simulink model "Symmetry"  (Simulink 8.3)
settings: Solver=ode23t  StartTime=0.0  StopTime=tfin  RelTol=1e-4
values from neighbouring files (symbols this model uses):
  Butterworth_filter_order = 8    [Sketch_controller_model_ini.m]    (also in Symmetry_ini.m; Symmetry_ini_COPY.m)
  C_Network = [0, 0, 0]    [Symmetry_ini.m]    (also in Symmetry_ini_COPY.m)
  Capacitive_Load_R_RC = [25,    50,   35;                                10e-3, 5e-3, 7e-3]    [Symmetry_ini.m]    (also in Symmetry_ini_COPY.m = [60e-3,  120e-3,  80e-3;                                1e-3)
  Capacitive_Load_R_Switching_Sequence = Capacitive_Load_R_Switching_Sequence_'    [Symmetry_ini.m]    (also in Symmetry_ini_COPY.m = ones(3,tfin/Capacitive_Load_R_Switching_Speed(1))')
  Capacitive_Load_R_Switching_Speed = [0.02,0.02,0.02]    [Symmetry_ini.m]    (also in Symmetry_ini_COPY.m = [0.01,0.01,0.01])
  Capacitive_Load_S_RC = [25,    50,   35;                                10e-3, 5e-3, 7e-3]    [Symmetry_ini.m]    (also in Symmetry_ini_COPY.m = [60e-3,  120e-3,  80e-3;                                1e-3)
  Capacitive_Load_S_Switching_Sequence = Capacitive_Load_S_Switching_Sequence_'    [Symmetry_ini.m]    (also in Symmetry_ini_COPY.m = ones(3,tfin/Capacitive_Load_R_Switching_Speed(1))')
  Capacitive_Load_S_Switching_Speed = [0.01,0.01,0.01]    [Symmetry_ini.m]    (also in Symmetry_ini_COPY.m)
  Capacitive_Load_T_RC = [25,    50,   35;                                10e-3, 5e-3, 7e-3]    [Symmetry_ini.m]    (also in Symmetry_ini_COPY.m = [60e-3,  120e-3,  80e-3;                                1e-3)
  Capacitive_Load_T_Switching_Sequence = Capacitive_Load_T_Switching_Sequence_'    [Symmetry_ini.m]    (also in Symmetry_ini_COPY.m = ones(3,tfin/Capacitive_Load_R_Switching_Speed(1))')
  Capacitive_Load_T_Switching_Speed = [0.01,0.01,0.01]    [Symmetry_ini.m]    (also in Symmetry_ini_COPY.m)
  i = str2num(answer{1})/sample    [Test_intersect.m]
  Inductive_Load_Switching_Sequence = Inductive_Load_Switching_Sequence_'    [Symmetry_ini.m]    (also in Symmetry_ini_COPY.m = ones(3,tfin/Inductive_Load_Switching_Speed(1))')
  Inductive_Load_Switching_Speed = [0.01,0.01,0.01]    [Symmetry_ini.m]    (also in Symmetry_ini_COPY.m)
  L_Network = [3.185e-3, 3.185e-3, 3.185e-3, 3.185e-3]    [Symmetry_ini.m]    (also in Symmetry_ini_COPY.m)
  L_Source = [3.185e-3, 3.185e-3, 3.185e-3]    [Sketch_controller_model_ini.m]    (also in Symmetry_ini.m; Symmetry_ini_COPY.m)
  Load_R = [50,50,50]    [Symmetry_ini.m]    (also in Symmetry_ini_COPY.m)
  Load_RL = [35.35,   35.35,   35.35;                  0.1125,  0.1125,  0.1125]    [Symmetry_ini.m]    (also in Symmetry_ini_COPY.m)
  Load_Wire_Resistance = [0.1,0.2]    [Symmetry_ini.m]    (also in Symmetry_ini_COPY.m)
  Ohmic_Load_Switching_Sequence = Ohmic_Load_Switching_Sequence_'    [Symmetry_ini.m]    (also in Symmetry_ini_COPY.m = ones(3,tfin/Ohmic_Load_Switching_Speed(1))')
  Ohmic_Load_Switching_Speed = [0.01,0.01,0.01]    [Symmetry_ini.m]    (also in Symmetry_ini_COPY.m)
  Phase_Source = [0,2/3*pi,4/3*pi]    [Sketch_controller_model_ini.m]    (also in Symmetry_REAL_TIME_ini.m = [0,-2/3*pi,-4/3*pi]; Symmetry_ini.m; Symmetry_ini_COPY.m = [0,-2/3*pi,-4/3*pi])
  R_Network = [0.4, 0.4, 0.4, 0.4]    [Symmetry_ini.m]    (also in Symmetry_ini_COPY.m)
  R_Source = [0.4, 0.4, 0.4]    [Sketch_controller_model_ini.m]    (also in Symmetry_ini.m; Symmetry_ini_COPY.m)
  sample = 10e-5    (= 0.0001)    [Inverter_ini.m]    (also in Sketch_controller_model_ini.m; Symmetry_REAL_TIME_ini.m; Symmetry_ini.m; Symmetry_ini_COPY.m)
  Source_Frequency = [50,50,50]    [Sketch_controller_model_ini.m]    (also in Symmetry_ini.m; Symmetry_ini_COPY.m)
  Switch_Load_R = [1,1,1]    [Symmetry_ini.m]    (also in Symmetry_ini_COPY.m = [1,0,0])
  Switch_Load_RC = [1,1,1]    [Symmetry_ini.m]    (also in Symmetry_ini_COPY.m = [0,0,1])
  Switch_Load_RL = [1,1,1]    [Symmetry_ini.m]    (also in Symmetry_ini_COPY.m = [0,1,0])
  Urms_Source = [230,230,230]    [Sketch_controller_model_ini.m]    (also in Symmetry_REAL_TIME_ini.m; Symmetry_ini.m; Symmetry_ini_COPY.m)
libraries: powerlib x87, simulink x15, powerlib_extras x12, dsparch4 x3
settings Model: Creator=gorbep  LastModifiedBy=Templomos
settings SolverCC: ZeroCrossControl=EnableAll  ZeroCrossAlgorithm=Adaptive  SolverResetMethod=Robust
settings DataIOCC: SignalLoggingSaveFormat=Dataset
settings DebuggingCC: UnderspecifiedInitializationDetection=Simplified  StateNameClashWarn=none
settings GRTTargetCC: CombineOutputUpdateFcns=on  GRTInterface=off

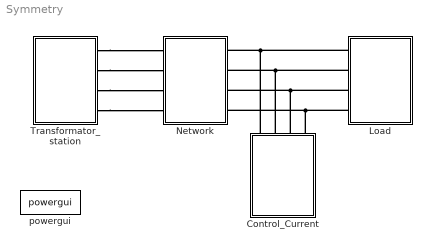
== system Symmetry ==
  Control_Current : Subsystem
  Load : Subsystem
  Network : Subsystem
  Transformator_station : Subsystem
  powergui : powerlib/powergui  SimulationMode=Continuous  SolverType=Tustin  SampleTime=50e-6  frequency=60  SPID=off  DisableSnubberDevices=off  DisableRonSwitches=off  DisableVfSwitches=off  SwTol=0  Interpol=off  DisplayEquations=off  Ts=0  methode=off  frequencyindice=0  Pbase=100e6  ErrMax=1e-4  Iterations=50  UnitsV=kV  UnitsW=MW  FunctionMessages=off  echomessages=off  HookPort=off  EnableUseOfTLC=off  x0status=blocks  RestoreLinks=warning  ResistiveCurrentMeasurement=off  Frange=[0:2:500]  Ylog=off  Xlog=on  ShowGrid=off  save=off  variable=ZData  structure=0  ZoomFFT=on  StartTime=0.0  cycles=1  DisplayStyle=1  fundamental=60  FreqAxis=off  MaxFrequency=1000  frequencyindicesteady=1  RmsSteady=1  display=off
  connections:
  Transformator_station/RConn1 -- Network/LConn1
  Transformator_station/RConn2 -- Network/LConn2
  Transformator_station/RConn3 -- Network/LConn3
  Transformator_station/RConn4 -- Network/LConn4
  Load/LConn1 -- Control_Current/RConn1 -- Network/RConn1
  Load/LConn2 -- Control_Current/RConn2 -- Network/RConn2
  Load/LConn3 -- Control_Current/RConn3 -- Network/RConn3
  Load/LConn4 -- Control_Current/RConn4 -- Network/RConn4

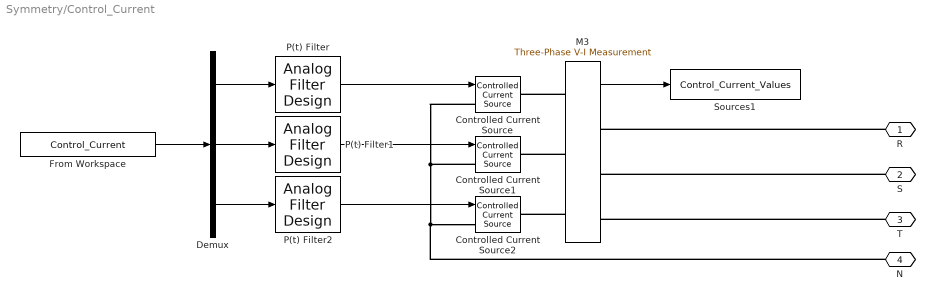
== system Symmetry/Control_Current ==
  Controlled Current Source : powerlib/Electrical Sources/Controlled Current Source  Initialize=on  Source_Type=AC  Amplitude=0  Phase=0  Frequency=0  Measurements=None
  Controlled Current Source1 : powerlib/Electrical Sources/Controlled Current Source  Initialize=on  Source_Type=AC  Amplitude=0  Phase=0  Frequency=0  Measurements=None
  Controlled Current Source2 : powerlib/Electrical Sources/Controlled Current Source  Initialize=on  Source_Type=AC  Amplitude=0  Phase=0  Frequency=0  Measurements=None
  Demux : Demux  Outputs=3
  From Workspace : FromWorkspace  VariableName=Control_Current  OutDataTypeStr=double  SampleTime=sample
  M3 : powerlib/Measurements/Three-Phase V-I Measurement  VoltageMeasurement=no  SetLabelV=off  LabelV=V_RST  Vpu=off  VpuLL=off  CurrentMeasurement=yes  SetLabelI=off  LabelI=I_RST  Ipu=off  Pbase=100e6  Vbase=500e3  OutputType=Complex  PhasorSimulation=off  PSBequivalent=0
  P(t) Filter : dsparch4/Analog Filter Design  method=Butterworth  filttype=Lowpass  N=Butterworth_filter_order  Wlo=Butterworth_passband_frequency  Whi=80  Rp=2  Rs=40
  P(t) Filter1 : dsparch4/Analog Filter Design  method=Butterworth  filttype=Lowpass  N=Butterworth_filter_order  Wlo=Butterworth_passband_frequency  Whi=80  Rp=2  Rs=40
  P(t) Filter2 : dsparch4/Analog Filter Design  method=Butterworth  filttype=Lowpass  N=Butterworth_filter_order  Wlo=Butterworth_passband_frequency  Whi=80  Rp=2  Rs=40
  Sources1 : ToWorkspace  VariableName=Control_Current_Values  SaveFormat=Structure With Time  SampleTime=sample
  R : PMIOPort  Port=1  Side=Right
  S : PMIOPort  Port=2  Side=Right
  T : PMIOPort  Port=3  Side=Right
  N : PMIOPort  Port=4  Side=Right
  wires:
  From Workspace/1 -> Demux/1
  M3/1 -> Sources1/1
  P(t) Filter2/1 -> Controlled Current Source2/1
  Demux/1 -> P(t) Filter/1
  Demux/2 -> P(t) Filter1/1
  P(t) Filter1/1 -> Controlled Current Source1/1
  P(t) Filter/1 -> Controlled Current Source/1
  Demux/3 -> P(t) Filter2/1
  connections:
  Controlled Current Source/LConn1 -- Controlled Current Source1/LConn1 -- Controlled Current Source2/LConn1 -- N/RConn1
  M3/LConn1 -- Controlled Current Source/RConn1
  M3/LConn2 -- Controlled Current Source1/RConn1
  M3/LConn3 -- Controlled Current Source2/RConn1
  R/RConn1 -- M3/RConn1
  S/RConn1 -- M3/RConn2
  T/RConn1 -- M3/RConn3

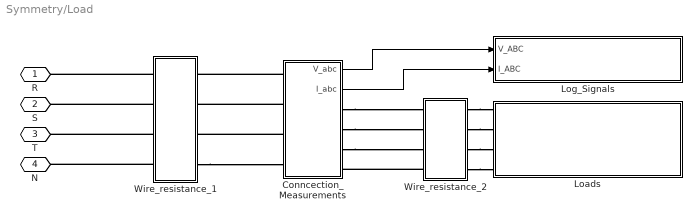
== system Symmetry/Load ==
  Conncection_Measurements : Subsystem
  Loads : Subsystem
  Log_Signals : Subsystem
  Wire_resistance_1 : Subsystem
  Wire_resistance_2 : Subsystem
  R : PMIOPort  Port=1  Side=Left
  S : PMIOPort  Port=2  Side=Left
  T : PMIOPort  Port=3  Side=Left
  N : PMIOPort  Port=4  Side=Left
  wires:
  Conncection_Measurements/2(I_abc) -> Log_Signals/2(I_ABC)
  Conncection_Measurements/1(V_abc) -> Log_Signals/1(V_ABC)
  connections:
  Conncection_Measurements/RConn1 -- Wire_resistance_2/LConn1
  Conncection_Measurements/RConn2 -- Wire_resistance_2/LConn2
  Conncection_Measurements/RConn3 -- Wire_resistance_2/LConn3
  Wire_resistance_1/LConn1 -- R/RConn1
  Wire_resistance_1/LConn2 -- S/RConn1
  Wire_resistance_1/LConn3 -- T/RConn1
  Wire_resistance_1/LConn4 -- N/RConn1
  Conncection_Measurements/LConn1 -- Wire_resistance_1/RConn1
  Conncection_Measurements/LConn2 -- Wire_resistance_1/RConn2
  Conncection_Measurements/LConn3 -- Wire_resistance_1/RConn3
  Wire_resistance_2/RConn1 -- Loads/LConn1
  Wire_resistance_2/RConn2 -- Loads/LConn2
  Wire_resistance_2/RConn3 -- Loads/LConn3
  Wire_resistance_2/RConn4 -- Loads/LConn4
  Wire_resistance_1/RConn4 -- Conncection_Measurements/LConn4
  Wire_resistance_2/LConn4 -- Conncection_Measurements/RConn4

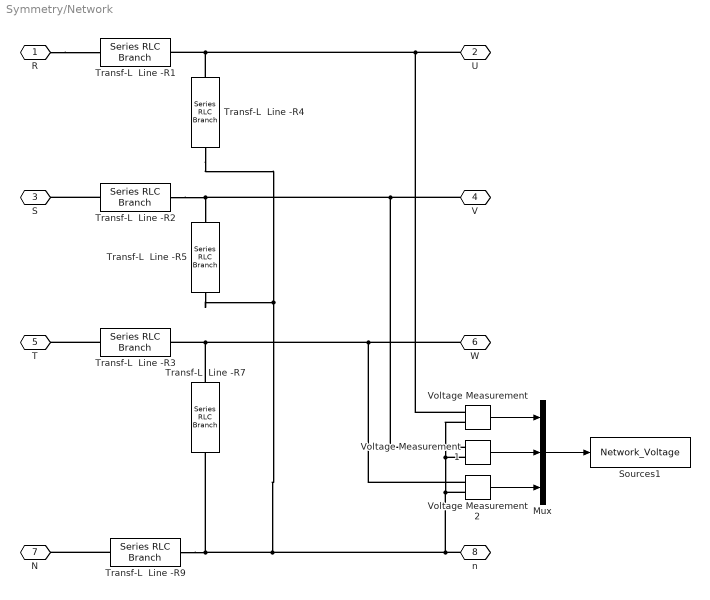
== system Symmetry/Network ==
  Mux : Mux  Inputs=3
  Sources1 : ToWorkspace  VariableName=Network_Voltage  SaveFormat=Structure With Time  SampleTime=-1
  Transf-L  Line -R1 : powerlib/Elements/Series RLC Branch  LConnTagsString=__new0  RConnTagsString=__new0  BranchType=RL  Resistance=R_Network(1)  Inductance=L_Network(1)  SetiL0=off  InitialCurrent=0  Capacitance=1.0  Setx0=off  InitialVoltage=0  Measurements=None
  Transf-L  Line -R2 : powerlib/Elements/Series RLC Branch  LConnTagsString=__new0  RConnTagsString=__new0  BranchType=RL  Resistance=R_Network(2)  Inductance=L_Network(2)  SetiL0=off  InitialCurrent=0  Capacitance=1.0  Setx0=off  InitialVoltage=0  Measurements=None
  Transf-L  Line -R3 : powerlib/Elements/Series RLC Branch  LConnTagsString=__new0  RConnTagsString=__new0  BranchType=RL  Resistance=R_Network(3)  Inductance=L_Network(3)  SetiL0=off  InitialCurrent=0  Capacitance=1.0  Setx0=off  InitialVoltage=0  Measurements=None
  Transf-L  Line -R4 : powerlib/Elements/Series RLC Branch  LConnTagsString=__new0  RConnTagsString=__new0  BranchType=C  Resistance=i  Inductance=0.003185  SetiL0=off  InitialCurrent=0  Capacitance=C_Network(1)  Setx0=off  InitialVoltage=0  Measurements=None
  Transf-L  Line -R5 : powerlib/Elements/Series RLC Branch  LConnTagsString=__new0  RConnTagsString=__new0  BranchType=C  Resistance=i  Inductance=0.003185  SetiL0=off  InitialCurrent=0  Capacitance=C_Network(2)  Setx0=off  InitialVoltage=0  Measurements=None
  Transf-L  Line -R7 : powerlib/Elements/Series RLC Branch  LConnTagsString=__new0  RConnTagsString=__new0  BranchType=C  Resistance=i  Inductance=0.003185  SetiL0=off  InitialCurrent=0  Capacitance=C_Network(2)  Setx0=off  InitialVoltage=0  Measurements=None
  Transf-L  Line -R9 : powerlib/Elements/Series RLC Branch  LConnTagsString=__new0  RConnTagsString=__new0  BranchType=RL  Resistance=R_Network(4)  Inductance=L_Network(4)  SetiL0=off  InitialCurrent=0  Capacitance=1.0  Setx0=off  InitialVoltage=0  Measurements=None
  Voltage Measurement : powerlib/Measurements/Voltage Measurement  PhasorSimulation=off  OutputType=Complex  PSBequivalent=0
  Voltage Measurement1 : powerlib/Measurements/Voltage Measurement  PhasorSimulation=off  OutputType=Complex  PSBequivalent=0
  Voltage Measurement2 : powerlib/Measurements/Voltage Measurement  PhasorSimulation=off  OutputType=Complex  PSBequivalent=0
  R : PMIOPort  Port=1  Side=Left
  U : PMIOPort  Port=2  Side=Right
  S : PMIOPort  Port=3  Side=Left
  V : PMIOPort  Port=4  Side=Right
  T : PMIOPort  Port=5  Side=Left
  W : PMIOPort  Port=6  Side=Right
  N : PMIOPort  Port=7  Side=Left
  n : PMIOPort  Port=8  Side=Right
  wires:
  Voltage Measurement/1 -> Mux/1
  Voltage Measurement1/1 -> Mux/2
  Voltage Measurement2/1 -> Mux/3
  Mux/1 -> Sources1/1
  connections:
  Transf-L  Line -R4/LConn1 -- Voltage Measurement/LConn1 -- U/RConn1 -- Transf-L  Line -R1/RConn1
  Transf-L  Line -R2/RConn1 -- Voltage Measurement1/LConn1 -- V/RConn1 -- Transf-L  Line -R5/LConn1
  Transf-L  Line -R7/LConn1 -- Voltage Measurement2/LConn1 -- W/RConn1 -- Transf-L  Line -R3/RConn1
  Transf-L  Line -R3/LConn1 -- T/RConn1
  Transf-L  Line -R2/LConn1 -- S/RConn1
  R/RConn1 -- Transf-L  Line -R1/LConn1
  Voltage Measurement/LConn2 -- Voltage Measurement1/LConn2 -- Transf-L  Line -R7/RConn1 -- Transf-L  Line -R9/RConn1 -- Transf-L  Line -R4/RConn1 -- Transf-L  Line -R5/RConn1 -- n/RConn1 -- Voltage Measurement2/LConn2
  Transf-L  Line -R9/LConn1 -- N/RConn1

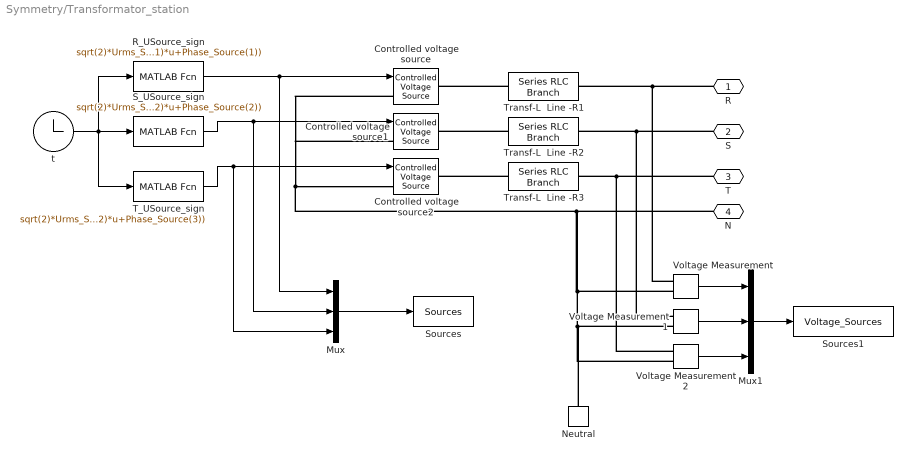
== system Symmetry/Transformator_station ==
  " R_USource_sign" : MATLABFcn  MATLABFcn=sqrt(2)*Urms_Source(1)*sin(2*pi*Source_Frequency(1)*u+Phase_Source(1))  SampleTime=sample
  " S_USource_sign" : MATLABFcn  MATLABFcn=sqrt(2)*Urms_Source(2)*sin(2*pi*Source_Frequency(2)*u+Phase_Source(2))  SampleTime=sample
  " T_USource_sign" : MATLABFcn  MATLABFcn=sqrt(2)*Urms_Source(3)*sin(2*pi*Source_Frequency(2)*u+Phase_Source(3))  SampleTime=sample
  Controlled voltage source : powerlib/Electrical Sources/Controlled Voltage Source  Initialize=off  Source_Type=AC  Amplitude=0  Phase=0  Frequency=0  Measurements=None
  Controlled voltage source1 : powerlib/Electrical Sources/Controlled Voltage Source  Initialize=off  Source_Type=AC  Amplitude=0  Phase=0  Frequency=0  Measurements=None
  Controlled voltage source2 : powerlib/Electrical Sources/Controlled Voltage Source  Initialize=off  Source_Type=AC  Amplitude=0  Phase=0  Frequency=0  Measurements=None
  Mux : Mux  Inputs=3
  Mux1 : Mux  Inputs=3
  Neutral : powerlib/Elements/Neutral  LConnTagsString=a  NodeNumber=10
  Sources : ToWorkspace  VariableName=Sources  SaveFormat=Structure With Time  SampleTime=-1
  Sources1 : ToWorkspace  VariableName=Voltage_Sources  SaveFormat=Structure With Time  SampleTime=-1
  Transf-L  Line -R1 : powerlib/Elements/Series RLC Branch  LConnTagsString=__new0  RConnTagsString=__new0  BranchType=RL  Resistance=R_Source(1)  Inductance=L_Source(1)  SetiL0=off  InitialCurrent=0  Capacitance=1.0  Setx0=off  InitialVoltage=0  Measurements=None
  Transf-L  Line -R2 : powerlib/Elements/Series RLC Branch  LConnTagsString=__new0  RConnTagsString=__new0  BranchType=RL  Resistance=R_Source(2)  Inductance=L_Source(2)  SetiL0=off  InitialCurrent=0  Capacitance=1.0  Setx0=off  InitialVoltage=0  Measurements=None
  Transf-L  Line -R3 : powerlib/Elements/Series RLC Branch  LConnTagsString=__new0  RConnTagsString=__new0  BranchType=RL  Resistance=R_Source(3)  Inductance=L_Source(3)  SetiL0=off  InitialCurrent=0  Capacitance=1.0  Setx0=off  InitialVoltage=0  Measurements=None
  Voltage Measurement : powerlib/Measurements/Voltage Measurement  PhasorSimulation=off  OutputType=Complex  PSBequivalent=0
  Voltage Measurement1 : powerlib/Measurements/Voltage Measurement  PhasorSimulation=off  OutputType=Complex  PSBequivalent=0
  Voltage Measurement2 : powerlib/Measurements/Voltage Measurement  PhasorSimulation=off  OutputType=Complex  PSBequivalent=0
  t : Clock
      settings: Decimation=CLK
  R : PMIOPort  Port=1  Side=Right
  S : PMIOPort  Port=2  Side=Right
  T : PMIOPort  Port=3  Side=Right
  N : PMIOPort  Port=4  Side=Right
  wires:
  Mux/1 -> Sources/1
  " R_USource_sign"/1 -> Mux/1, Controlled voltage source/1
  " S_USource_sign"/1 -> Mux/2, Controlled voltage source1/1
  " T_USource_sign"/1 -> Mux/3, Controlled voltage source2/1
  t/1 -> " R_USource_sign"/1, " T_USource_sign"/1, " S_USource_sign"/1
  Voltage Measurement/1 -> Mux1/1
  Voltage Measurement1/1 -> Mux1/2
  Voltage Measurement2/1 -> Mux1/3
  Mux1/1 -> Sources1/1
  connections:
  N/RConn1 -- Neutral/LConn1 -- Voltage Measurement2/LConn2 -- Voltage Measurement1/LConn2 -- Voltage Measurement/LConn2 -- Controlled voltage source/LConn1 -- Controlled voltage source1/LConn1 -- Controlled voltage source2/LConn1
  Transf-L  Line -R2/LConn1 -- Controlled voltage source1/RConn1
  Transf-L  Line -R3/LConn1 -- Controlled voltage source2/RConn1
  Transf-L  Line -R1/LConn1 -- Controlled voltage source/RConn1
  R/RConn1 -- Voltage Measurement/LConn1 -- Transf-L  Line -R1/RConn1
  S/RConn1 -- Voltage Measurement1/LConn1 -- Transf-L  Line -R2/RConn1
  T/RConn1 -- Voltage Measurement2/LConn1 -- Transf-L  Line -R3/RConn1

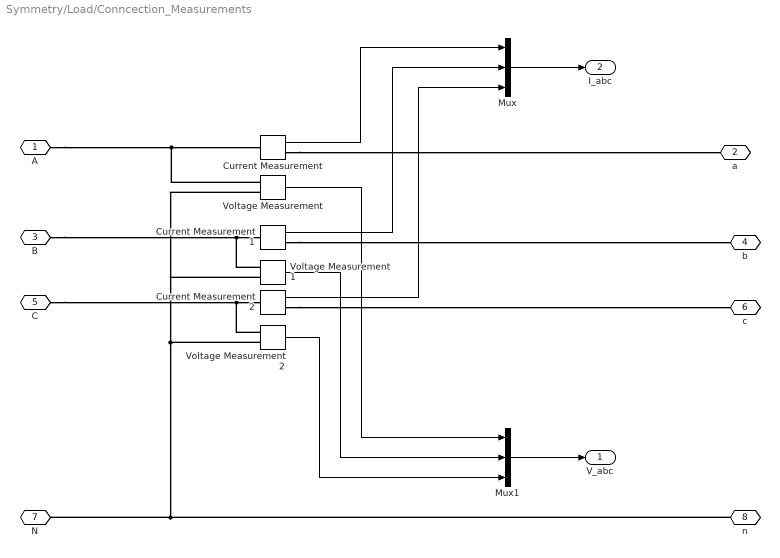
== system Symmetry/Load/Conncection_Measurements ==
  Current Measurement : powerlib/Measurements/Current Measurement  PhasorSimulation=off  OutputType=Complex  PSBequivalent=0
  Current Measurement1 : powerlib/Measurements/Current Measurement  PhasorSimulation=off  OutputType=Complex  PSBequivalent=0
  Current Measurement2 : powerlib/Measurements/Current Measurement  PhasorSimulation=off  OutputType=Complex  PSBequivalent=0
  Mux : Mux  Inputs=3
  Mux1 : Mux  Inputs=3
  Voltage Measurement : powerlib/Measurements/Voltage Measurement  PhasorSimulation=off  OutputType=Complex  PSBequivalent=0
  Voltage Measurement1 : powerlib/Measurements/Voltage Measurement  PhasorSimulation=off  OutputType=Complex  PSBequivalent=0
  Voltage Measurement2 : powerlib/Measurements/Voltage Measurement  PhasorSimulation=off  OutputType=Complex  PSBequivalent=0
  A : PMIOPort  Port=1  Side=Left
  a : PMIOPort  Port=2  Side=Right
  B : PMIOPort  Port=3  Side=Left
  b : PMIOPort  Port=4  Side=Right
  C : PMIOPort  Port=5  Side=Left
  c : PMIOPort  Port=6  Side=Right
  N : PMIOPort  Port=7  Side=Left
  n : PMIOPort  Port=8  Side=Right
  V_abc : Outport
  I_abc : Outport  Port=2
  wires:
  Current Measurement1/1 -> Mux/2
  Mux1/1 -> V_abc/1
  Mux/1 -> I_abc/1
  Current Measurement/1 -> Mux/1
  Voltage Measurement/1 -> Mux1/1
  Current Measurement2/1 -> Mux/3
  Voltage Measurement1/1 -> Mux1/2
  Voltage Measurement2/1 -> Mux1/3
  connections:
  Current Measurement2/RConn1 -- c/RConn1
  Current Measurement/RConn1 -- a/RConn1
  Current Measurement1/RConn1 -- b/RConn1
  Voltage Measurement2/LConn1 -- Current Measurement2/LConn1 -- C/RConn1
  Voltage Measurement2/LConn2 -- N/RConn1 -- n/RConn1 -- Voltage Measurement1/LConn2 -- Voltage Measurement/LConn2
  Voltage Measurement1/LConn1 -- Current Measurement1/LConn1 -- B/RConn1
  Voltage Measurement/LConn1 -- A/RConn1 -- Current Measurement/LConn1

== system Symmetry/Load/Loads ==
  Capacitive_Loads_RST : Subsystem
  Inductive_Loads_RST : Subsystem
  Ohmic_Loads_RST : Subsystem
  R : PMIOPort  Port=1  Side=Left
  S : PMIOPort  Port=2  Side=Left
  T : PMIOPort  Port=3  Side=Left
  N : PMIOPort  Port=4  Side=Left
  connections:
  Ohmic_Loads_RST/LConn1 -- R/RConn1 -- Inductive_Loads_RST/LConn1 -- Capacitive_Loads_RST/RConn1
  Capacitive_Loads_RST/RConn2 -- S/RConn1 -- Inductive_Loads_RST/LConn2 -- Ohmic_Loads_RST/LConn2
  Capacitive_Loads_RST/RConn3 -- T/RConn1 -- Inductive_Loads_RST/LConn3 -- Ohmic_Loads_RST/LConn3
  N/RConn1 -- Inductive_Loads_RST/RConn1 -- Ohmic_Loads_RST/RConn1 -- Capacitive_Loads_RST/LConn1

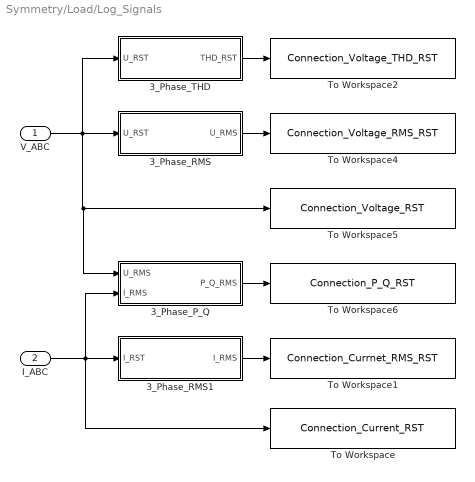
== system Symmetry/Load/Log_Signals ==
  V_ABC : Inport
  I_ABC : Inport  Port=2
  3_Phase_P_Q : Subsystem
  3_Phase_RMS : Subsystem
  3_Phase_RMS1 : Subsystem
  3_Phase_THD : Subsystem
  To Workspace : ToWorkspace  VariableName=Connection_Current_RST  SaveFormat=Timeseries  SampleTime=sample
  To Workspace1 : ToWorkspace  VariableName=Connection_Currnet_RMS_RST  SaveFormat=Timeseries  SampleTime=sample
  To Workspace2 : ToWorkspace  VariableName=Connection_Voltage_THD_RST  SaveFormat=Timeseries  SampleTime=sample
  To Workspace4 : ToWorkspace  VariableName=Connection_Voltage_RMS_RST  SaveFormat=Timeseries  SampleTime=sample
  To Workspace5 : ToWorkspace  VariableName=Connection_Voltage_RST  SaveFormat=Timeseries  SampleTime=sample
  To Workspace6 : ToWorkspace  VariableName=Connection_P_Q_RST  SaveFormat=Timeseries  SampleTime=sample
  wires:
  I_ABC/1 -> 3_Phase_RMS1/1(I_RST), To Workspace/1, 3_Phase_P_Q/2(I_RMS)
  V_ABC/1 -> 3_Phase_RMS/1(U_RST), 3_Phase_THD/1(U_RST), To Workspace5/1, 3_Phase_P_Q/1(U_RMS)
  3_Phase_RMS1/1(I_RMS) -> To Workspace1/1
  3_Phase_RMS/1(U_RMS) -> To Workspace4/1
  3_Phase_P_Q/1(P_Q_RMS) -> To Workspace6/1
  3_Phase_THD/1(THD_RST) -> To Workspace2/1

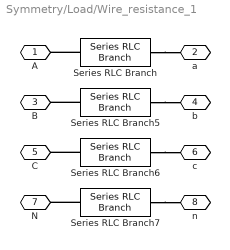
== system Symmetry/Load/Wire_resistance_1 ==
  Series RLC Branch{,5..7} (4 alike) : powerlib/Elements/Series RLC Branch  LConnTagsString=__new0  RConnTagsString=__new0  BranchType=R  Resistance=Load_Wire_Resistance(1)  Inductance=1e-3  SetiL0=off  InitialCurrent=0  Capacitance=1e-6  Setx0=off  InitialVoltage=0  Measurements=None
  A : PMIOPort  Port=1  Side=Left
  a : PMIOPort  Port=2  Side=Right
  B : PMIOPort  Port=3  Side=Left
  b : PMIOPort  Port=4  Side=Right
  C : PMIOPort  Port=5  Side=Left
  c : PMIOPort  Port=6  Side=Right
  N : PMIOPort  Port=7  Side=Left
  n : PMIOPort  Port=8  Side=Right
  connections:
  Series RLC Branch7/RConn1 -- n/RConn1
  Series RLC Branch5/LConn1 -- B/RConn1
  Series RLC Branch6/LConn1 -- C/RConn1
  Series RLC Branch/RConn1 -- a/RConn1
  Series RLC Branch/LConn1 -- A/RConn1
  Series RLC Branch7/LConn1 -- N/RConn1
  Series RLC Branch6/RConn1 -- c/RConn1
  Series RLC Branch5/RConn1 -- b/RConn1

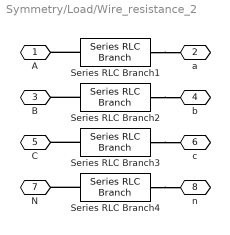
== system Symmetry/Load/Wire_resistance_2 ==
  Series RLC Branch{1..4} (4 alike) : powerlib/Elements/Series RLC Branch  LConnTagsString=__new0  RConnTagsString=__new0  BranchType=R  Resistance=Load_Wire_Resistance(2)  Inductance=1e-3  SetiL0=off  InitialCurrent=0  Capacitance=1e-6  Setx0=off  InitialVoltage=0  Measurements=None
  A : PMIOPort  Port=1  Side=Left
  a : PMIOPort  Port=2  Side=Right
  B : PMIOPort  Port=3  Side=Left
  b : PMIOPort  Port=4  Side=Right
  C : PMIOPort  Port=5  Side=Left
  c : PMIOPort  Port=6  Side=Right
  N : PMIOPort  Port=7  Side=Left
  n : PMIOPort  Port=8  Side=Right
  connections:
  Series RLC Branch2/RConn1 -- b/RConn1
  Series RLC Branch1/RConn1 -- a/RConn1
  Series RLC Branch4/RConn1 -- n/RConn1
  Series RLC Branch2/LConn1 -- B/RConn1
  Series RLC Branch3/RConn1 -- c/RConn1
  Series RLC Branch3/LConn1 -- C/RConn1
  Series RLC Branch1/LConn1 -- A/RConn1
  Series RLC Branch4/LConn1 -- N/RConn1

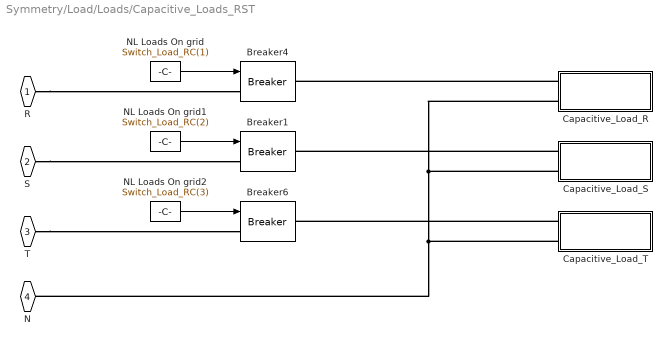
== system Symmetry/Load/Loads/Capacitive_Loads_RST ==
  Breaker1 : powerlib/Elements/Breaker  InitialState=0  SwitchingTimes="[ 1/60  5/60 ]"  External=on  BreakerResistance=0.01  SnubberResistance=1e7  SnubberCapacitance=inf  Measurements=None  MoreParameters=off  NoBreakLoop=off
  Breaker4 : powerlib/Elements/Breaker  InitialState=0  SwitchingTimes="[ 1/60  5/60 ]"  External=on  BreakerResistance=0.01  SnubberResistance=1e7  SnubberCapacitance=inf  Measurements=None  MoreParameters=off  NoBreakLoop=off
  Breaker6 : powerlib/Elements/Breaker  InitialState=0  SwitchingTimes="[ 1/60  5/60 ]"  External=on  BreakerResistance=0.01  SnubberResistance=1e7  SnubberCapacitance=inf  Measurements=None  MoreParameters=off  NoBreakLoop=off
  Capacitive_Load_R : Subsystem
  Capacitive_Load_S : Subsystem
  Capacitive_Load_T : Subsystem
  NL Loads On grid : Constant  Value=Switch_Load_RC(1)
  NL Loads On grid1 : Constant  Value=Switch_Load_RC(2)
  NL Loads On grid2 : Constant  Value=Switch_Load_RC(3)
  R : PMIOPort  Port=1  Side=Right
  S : PMIOPort  Port=2  Side=Right
  T : PMIOPort  Port=3  Side=Right
  N : PMIOPort  Port=4  Side=Left
  wires:
  NL Loads On grid/1 -> Breaker4/1
  NL Loads On grid1/1 -> Breaker1/1
  NL Loads On grid2/1 -> Breaker6/1
  connections:
  R/RConn1 -- Breaker4/LConn1
  S/RConn1 -- Breaker1/LConn1
  T/RConn1 -- Breaker6/LConn1
  Capacitive_Load_R/LConn1 -- Breaker4/RConn1
  Capacitive_Load_S/LConn1 -- Breaker1/RConn1
  Capacitive_Load_T/LConn1 -- Breaker6/RConn1
  Capacitive_Load_R/LConn2 -- Capacitive_Load_S/LConn2 -- Capacitive_Load_T/LConn2 -- N/RConn1

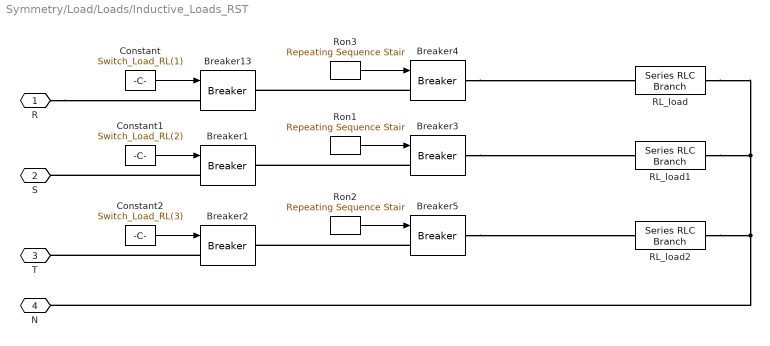
== system Symmetry/Load/Loads/Inductive_Loads_RST ==
  Breaker{1..5,13} (6 alike) : powerlib/Elements/Breaker  InitialState=0  SwitchingTimes="[ 1/60  5/60 ]"  External=on  BreakerResistance=0.01  SnubberResistance=1e7  SnubberCapacitance=inf  Measurements=None  MoreParameters=off  NoBreakLoop=off
  Constant : Constant  Value=Switch_Load_RL(1)
  Constant1 : Constant  Value=Switch_Load_RL(2)
  Constant2 : Constant  Value=Switch_Load_RL(3)
  RL_load : powerlib/Elements/Series RLC Branch  LConnTagsString=__new0  RConnTagsString=__new0  BranchType=RL  Resistance=Load_RL(1,1)  Inductance=Load_RL(2,1)  SetiL0=off  InitialCurrent=0  Capacitance=1.0  Setx0=off  InitialVoltage=0  Measurements=None
  RL_load1 : powerlib/Elements/Series RLC Branch  LConnTagsString=__new0  RConnTagsString=__new0  BranchType=RL  Resistance=Load_RL(1,2)  Inductance=Load_RL(2,2)  SetiL0=off  InitialCurrent=0  Capacitance=1.0  Setx0=off  InitialVoltage=0  Measurements=None
  RL_load2 : powerlib/Elements/Series RLC Branch  LConnTagsString=__new0  RConnTagsString=__new0  BranchType=RL  Resistance=Load_RL(1,3)  Inductance=Load_RL(2,3)  SetiL0=off  InitialCurrent=0  Capacitance=1.0  Setx0=off  InitialVoltage=0  Measurements=None
  Ron1 : simulink/Sources/Repeating Sequence Stair  OutValues=Inductive_Load_Switching_Sequence(:,2)  tsamp=Inductive_Load_Switching_Speed(2)  OutMin=[]  OutMax=[]  OutDataTypeStr=float('double')  OutputDataTypeScalingMode=Specify via dialog  OutDataType=float('double')  ConRadixGroup=Best Precision: Vector-wise  OutScaling=2^-12
  Ron2 : simulink/Sources/Repeating Sequence Stair  OutValues=Inductive_Load_Switching_Sequence(:,3)  tsamp=Inductive_Load_Switching_Speed(3)  OutMin=[]  OutMax=[]  OutDataTypeStr=float('double')  OutputDataTypeScalingMode=Specify via dialog  OutDataType=float('double')  ConRadixGroup=Best Precision: Vector-wise  OutScaling=2^-12
  Ron3 : simulink/Sources/Repeating Sequence Stair  OutValues=Inductive_Load_Switching_Sequence(:,1)  tsamp=Inductive_Load_Switching_Speed(1)  OutMin=[]  OutMax=[]  OutDataTypeStr=float('double')  OutputDataTypeScalingMode=Specify via dialog  OutDataType=float('double')  ConRadixGroup=Best Precision: Vector-wise  OutScaling=2^-12
  R : PMIOPort  Port=1  Side=Left
  S : PMIOPort  Port=2  Side=Left
  T : PMIOPort  Port=3  Side=Left
  N : PMIOPort  Port=4  Side=Right
  wires:
  Constant/1 -> Breaker13/1
  Constant1/1 -> Breaker1/1
  Constant2/1 -> Breaker2/1
  Ron3/1 -> Breaker4/1
  Ron1/1 -> Breaker3/1
  Ron2/1 -> Breaker5/1
  connections:
  RL_load/RConn1 -- RL_load1/RConn1 -- RL_load2/RConn1 -- N/RConn1
  R/RConn1 -- Breaker13/LConn1
  Breaker1/LConn1 -- S/RConn1
  Breaker2/LConn1 -- T/RConn1
  Breaker4/LConn1 -- Breaker13/RConn1
  Breaker3/LConn1 -- Breaker1/RConn1
  Breaker5/LConn1 -- Breaker2/RConn1
  Breaker4/RConn1 -- RL_load/LConn1
  Breaker3/RConn1 -- RL_load1/LConn1
  Breaker5/RConn1 -- RL_load2/LConn1

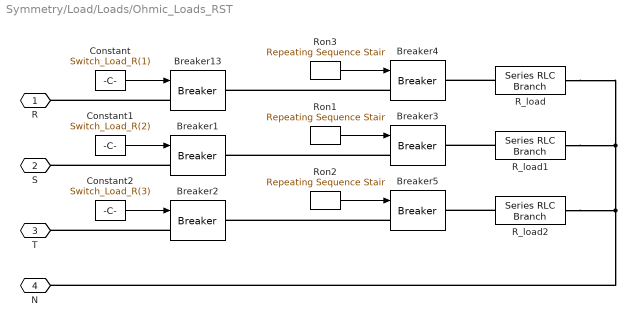
== system Symmetry/Load/Loads/Ohmic_Loads_RST ==
  Breaker{1..5,13} (6 alike) : powerlib/Elements/Breaker  InitialState=0  SwitchingTimes="[ 1/60  5/60 ]"  External=on  BreakerResistance=0.01  SnubberResistance=1e7  SnubberCapacitance=inf  Measurements=None  MoreParameters=off  NoBreakLoop=off
  Constant : Constant  Value=Switch_Load_R(1)
  Constant1 : Constant  Value=Switch_Load_R(2)
  Constant2 : Constant  Value=Switch_Load_R(3)
  R_load : powerlib/Elements/Series RLC Branch  LConnTagsString=__new0  RConnTagsString=__new0  BranchType=R  Resistance=Load_R(1)  Inductance=0.003185  SetiL0=off  InitialCurrent=0  Capacitance=1.0  Setx0=off  InitialVoltage=0  Measurements=None
  R_load1 : powerlib/Elements/Series RLC Branch  LConnTagsString=__new0  RConnTagsString=__new0  BranchType=R  Resistance=Load_R(2)  Inductance=0.003185  SetiL0=off  InitialCurrent=0  Capacitance=1.0  Setx0=off  InitialVoltage=0  Measurements=None
  R_load2 : powerlib/Elements/Series RLC Branch  LConnTagsString=__new0  RConnTagsString=__new0  BranchType=R  Resistance=Load_R(3)  Inductance=0.003185  SetiL0=off  InitialCurrent=0  Capacitance=1.0  Setx0=off  InitialVoltage=0  Measurements=None
  Ron1 : simulink/Sources/Repeating Sequence Stair  OutValues=Ohmic_Load_Switching_Sequence(:,2)  tsamp=Ohmic_Load_Switching_Speed(2)  OutMin=[]  OutMax=[]  OutDataTypeStr=float('double')  OutputDataTypeScalingMode=Specify via dialog  OutDataType=float('double')  ConRadixGroup=Best Precision: Vector-wise  OutScaling=2^-12
  Ron2 : simulink/Sources/Repeating Sequence Stair  OutValues=Ohmic_Load_Switching_Sequence(:,3)  tsamp=Ohmic_Load_Switching_Speed(3)  OutMin=[]  OutMax=[]  OutDataTypeStr=float('double')  OutputDataTypeScalingMode=Specify via dialog  OutDataType=float('double')  ConRadixGroup=Best Precision: Vector-wise  OutScaling=2^-12
  Ron3 : simulink/Sources/Repeating Sequence Stair  OutValues=Ohmic_Load_Switching_Sequence(:,1)  tsamp=Ohmic_Load_Switching_Speed(1)  OutMin=[]  OutMax=[]  OutDataTypeStr=float('double')  OutputDataTypeScalingMode=Specify via dialog  OutDataType=float('double')  ConRadixGroup=Best Precision: Vector-wise  OutScaling=2^-12
  R : PMIOPort  Port=1  Side=Left
  S : PMIOPort  Port=2  Side=Left
  T : PMIOPort  Port=3  Side=Left
  N : PMIOPort  Port=4  Side=Right
  wires:
  Constant/1 -> Breaker13/1
  Constant1/1 -> Breaker1/1
  Constant2/1 -> Breaker2/1
  Ron3/1 -> Breaker4/1
  Ron1/1 -> Breaker3/1
  Ron2/1 -> Breaker5/1
  connections:
  R_load/RConn1 -- R_load1/RConn1 -- R_load2/RConn1 -- N/RConn1
  Breaker13/LConn1 -- R/RConn1
  Breaker1/LConn1 -- S/RConn1
  Breaker2/LConn1 -- T/RConn1
  Breaker4/LConn1 -- Breaker13/RConn1
  Breaker3/LConn1 -- Breaker1/RConn1
  Breaker5/LConn1 -- Breaker2/RConn1
  R_load/LConn1 -- Breaker4/RConn1
  R_load1/LConn1 -- Breaker3/RConn1
  R_load2/LConn1 -- Breaker5/RConn1

== system Symmetry/Load/Log_Signals/3_Phase_P_Q ==
  U_RMS : Inport
  I_RMS : Inport  Port=2
  Demux1 : Demux  Outputs=3
  Demux3 : Demux  Outputs=3
  Mux4 : Mux  Inputs=3
  P Q in3 : powerlib_extras/Measurements/Active & Reactive Power  f1=Source_Frequency(1)
  P Q in4 : powerlib_extras/Measurements/Active & Reactive Power  f1=Source_Frequency(2)
  P Q in5 : powerlib_extras/Measurements/Active & Reactive Power  f1=Source_Frequency(3)
  P_Q_RMS : Outport
  wires:
  I_RMS/1 -> Demux1/1
  Demux1/3 -> P Q in5/2
  Demux1/2 -> P Q in4/2
  Demux1/1 -> P Q in3/2
  Demux3/3 -> P Q in5/1
  Demux3/2 -> P Q in4/1
  Demux3/1 -> P Q in3/1
  P Q in5/1 -> Mux4/3
  Mux4/1 -> P_Q_RMS/1
  U_RMS/1 -> Demux3/1
  P Q in4/1 -> Mux4/2
  P Q in3/1 -> Mux4/1

== system Symmetry/Load/Log_Signals/3_Phase_RMS ==
  U_RST : Inport
  Demux5 : Demux  Outputs=3
  Mux2 : Mux  Inputs=3
  RMS1 : powerlib_extras/Measurements/RMS  f1=Source_Frequency(2)
  RMS2 : powerlib_extras/Measurements/RMS  f1=Source_Frequency(3)
  RMS6 : powerlib_extras/Measurements/RMS  f1=Source_Frequency(1)
  U_RMS : Outport
  wires:
  RMS2/1 -> Mux2/3
  Demux5/2 -> RMS1/1
  U_RST/1 -> Demux5/1
  Demux5/3 -> RMS2/1
  RMS6/1 -> Mux2/1
  Demux5/1 -> RMS6/1
  RMS1/1 -> Mux2/2
  Mux2/1 -> U_RMS/1

== system Symmetry/Load/Log_Signals/3_Phase_RMS1 ==
  I_RST : Inport
  Demux5 : Demux  Outputs=3
  Mux2 : Mux  Inputs=3
  RMS1 : powerlib_extras/Measurements/RMS  f1=Source_Frequency(2)
  RMS2 : powerlib_extras/Measurements/RMS  f1=Source_Frequency(3)
  RMS6 : powerlib_extras/Measurements/RMS  f1=Source_Frequency(1)
  I_RMS : Outport
  wires:
  Demux5/3 -> RMS2/1
  Demux5/2 -> RMS1/1
  Demux5/1 -> RMS6/1
  Mux2/1 -> I_RMS/1
  RMS1/1 -> Mux2/2
  RMS6/1 -> Mux2/1
  I_RST/1 -> Demux5/1
  RMS2/1 -> Mux2/3

== system Symmetry/Load/Log_Signals/3_Phase_THD ==
  U_RST : Inport
  Demux1 : Demux  Outputs=3
  Mux7 : Mux  Inputs=3
  THD1 : powerlib_extras/Measurements/Total Harmonic Distortion  f1=Source_Frequency(2)
  THD2 : powerlib_extras/Measurements/Total Harmonic Distortion  f1=Source_Frequency(3)
  THD3 : powerlib_extras/Measurements/Total Harmonic Distortion  f1=Source_Frequency(1)
  THD_RST : Outport
  wires:
  THD1/1 -> Mux7/2
  THD2/1 -> Mux7/3
  THD3/1 -> Mux7/1
  Demux1/3 -> THD2/1
  Mux7/1 -> THD_RST/1
  U_RST/1 -> Demux1/1
  Demux1/2 -> THD1/1
  Demux1/1 -> THD3/1

== system Symmetry/Load/Loads/Capacitive_Loads_RST/Capacitive_Load_R ==
  Capacitive_Load_R_1 : Subsystem
  Capacitive_Load_R_2 : Subsystem
  Capacitive_Load_R_3 : Subsystem
  AC : PMIOPort  Port=1  Side=Left
  N : PMIOPort  Port=2  Side=Left
  connections:
  N/RConn1 -- Capacitive_Load_R_3/LConn2 -- Capacitive_Load_R_2/LConn2 -- Capacitive_Load_R_1/RConn2
  Capacitive_Load_R_2/LConn1 -- Capacitive_Load_R_1/RConn1 -- Capacitive_Load_R_3/LConn1 -- AC/RConn1

== system Symmetry/Load/Loads/Capacitive_Loads_RST/Capacitive_Load_S ==
  Capacitive_Load_S_1 : Subsystem
  Capacitive_Load_S_2 : Subsystem
  Capacitive_Load_S_3 : Subsystem
  AC : PMIOPort  Port=1  Side=Left
  N : PMIOPort  Port=2  Side=Left
  connections:
  AC/RConn1 -- Capacitive_Load_S_3/LConn1 -- Capacitive_Load_S_1/RConn1 -- Capacitive_Load_S_2/LConn1
  Capacitive_Load_S_1/RConn2 -- Capacitive_Load_S_2/LConn2 -- Capacitive_Load_S_3/LConn2 -- N/RConn1

== system Symmetry/Load/Loads/Capacitive_Loads_RST/Capacitive_Load_T ==
  Capacitive_Load_R_1 : Subsystem
  Capacitive_Load_R_2 : Subsystem
  Capacitive_Load_R_3 : Subsystem
  AC : PMIOPort  Port=1  Side=Left
  N : PMIOPort  Port=2  Side=Left
  connections:
  N/RConn1 -- Capacitive_Load_R_3/LConn2 -- Capacitive_Load_R_2/LConn2 -- Capacitive_Load_R_1/RConn2
  Capacitive_Load_R_2/LConn1 -- Capacitive_Load_R_1/RConn1 -- Capacitive_Load_R_3/LConn1 -- AC/RConn1

== system Symmetry/Load/Loads/Capacitive_Loads_RST/Capacitive_Load_R/Capacitive_Load_R_1 ==
  Breaker5 : powerlib/Elements/Breaker  InitialState=0  SwitchingTimes="[ 1/60  5/60 ]"  External=on  BreakerResistance=0.01  SnubberResistance=1e7  SnubberCapacitance=inf  Measurements=None  MoreParameters=off  NoBreakLoop=off
  Parallel RLC Branch : powerlib/Elements/Parallel RLC Branch  LConnTagsString=a  RConnTagsString=__new0  BranchType=RC  Resistance=Capacitive_Load_R_RC(1,1)  Inductance=1e-3  SetiL0=off  InitialCurrent=0  Capacitance=Capacitive_Load_R_RC(2,1)  Setx0=off  InitialVoltage=0  Measurements=None
  Ron3 : simulink/Sources/Repeating Sequence Stair  OutValues=Capacitive_Load_R_Switching_Sequence(:,1)  tsamp=Capacitive_Load_R_Switching_Speed(1)  OutMin=[]  OutMax=[]  OutDataTypeStr=float('double')  OutputDataTypeScalingMode=Specify via dialog  OutDataType=float('double')  ConRadixGroup=Best Precision: Vector-wise  OutScaling=2^-12
  Universal Bridge : powerlib/Power Electronics/Universal Bridge  Arms=2  SnubberResistance=1e5  SnubberCapacitance=inf  Device=Diodes  Ron=1e-3  Lon=0  ForwardVoltages="[  0  0  ]"  ForwardVoltage=0.8  GTOparameters=[ 10e-6 , 20e-6 ]  IGBTparameters=[ 1e-6 , 2e-6 ]  Measurements=None  Measurements_2=None  converterType=Rectifier
  AC : PMIOPort  Port=1  Side=Right
  N : PMIOPort  Port=2  Side=Right
  wires:
  Ron3/1 -> Breaker5/1
  connections:
  Universal Bridge/LConn2 -- N/RConn1
  Breaker5/RConn1 -- Universal Bridge/LConn1
  Universal Bridge/RConn1 -- Parallel RLC Branch/LConn1
  AC/RConn1 -- Breaker5/LConn1
  Universal Bridge/RConn2 -- Parallel RLC Branch/RConn1

== system Symmetry/Load/Loads/Capacitive_Loads_RST/Capacitive_Load_R/Capacitive_Load_R_2 ==
  Breaker2 : powerlib/Elements/Breaker  InitialState=0  SwitchingTimes="[ 1/60  5/60 ]"  External=on  BreakerResistance=0.01  SnubberResistance=1e7  SnubberCapacitance=inf  Measurements=None  MoreParameters=off  NoBreakLoop=off
  Parallel RLC Branch : powerlib/Elements/Parallel RLC Branch  LConnTagsString=a  RConnTagsString=__new0  BranchType=RC  Resistance=Capacitive_Load_R_RC(1,2)  Inductance=1e-3  SetiL0=off  InitialCurrent=0  Capacitance=Capacitive_Load_R_RC(2,2)  Setx0=off  InitialVoltage=0  Measurements=None
  Ron1 : simulink/Sources/Repeating Sequence Stair  OutValues=Capacitive_Load_R_Switching_Sequence(:,2)  tsamp=Capacitive_Load_R_Switching_Speed(2)  OutMin=[]  OutMax=[]  OutDataTypeStr=float('double')  OutputDataTypeScalingMode=Specify via dialog  OutDataType=float('double')  ConRadixGroup=Best Precision: Vector-wise  OutScaling=2^-12
  Universal Bridge1 : powerlib/Power Electronics/Universal Bridge  Arms=2  SnubberResistance=1e5  SnubberCapacitance=inf  Device=Diodes  Ron=1e-3  Lon=0  ForwardVoltages="[  0  0  ]"  ForwardVoltage=0.8  GTOparameters=[ 10e-6 , 20e-6 ]  IGBTparameters=[ 1e-6 , 2e-6 ]  Measurements=None  Measurements_2=None  converterType=Rectifier
  AC : PMIOPort  Port=1  Side=Left
  N : PMIOPort  Port=2  Side=Left
  wires:
  Ron1/1 -> Breaker2/1
  connections:
  Universal Bridge1/RConn2 -- Parallel RLC Branch/RConn1
  Universal Bridge1/LConn2 -- N/RConn1
  Breaker2/RConn1 -- Universal Bridge1/LConn1
  Parallel RLC Branch/LConn1 -- Universal Bridge1/RConn1
  AC/RConn1 -- Breaker2/LConn1

== system Symmetry/Load/Loads/Capacitive_Loads_RST/Capacitive_Load_R/Capacitive_Load_R_3 ==
  Breaker3 : powerlib/Elements/Breaker  InitialState=0  SwitchingTimes="[ 1/60  5/60 ]"  External=on  BreakerResistance=0.01  SnubberResistance=1e7  SnubberCapacitance=inf  Measurements=None  MoreParameters=off  NoBreakLoop=off
  Parallel RLC Branch : powerlib/Elements/Parallel RLC Branch  LConnTagsString=a  RConnTagsString=__new0  BranchType=RC  Resistance=Capacitive_Load_R_RC(1,3)  Inductance=1e-3  SetiL0=off  InitialCurrent=0  Capacitance=Capacitive_Load_R_RC(2,3)  Setx0=off  InitialVoltage=0  Measurements=None
  Ron4 : simulink/Sources/Repeating Sequence Stair  OutValues=Capacitive_Load_R_Switching_Sequence(:,3)  tsamp=Capacitive_Load_R_Switching_Speed(3)  OutMin=[]  OutMax=[]  OutDataTypeStr=float('double')  OutputDataTypeScalingMode=Specify via dialog  OutDataType=float('double')  ConRadixGroup=Best Precision: Vector-wise  OutScaling=2^-12
  Universal Bridge2 : powerlib/Power Electronics/Universal Bridge  Arms=2  SnubberResistance=1e5  SnubberCapacitance=inf  Device=Diodes  Ron=1e-3  Lon=0  ForwardVoltages="[  0  0  ]"  ForwardVoltage=0.8  GTOparameters=[ 10e-6 , 20e-6 ]  IGBTparameters=[ 1e-6 , 2e-6 ]  Measurements=None  Measurements_2=None  converterType=Rectifier
  AC : PMIOPort  Port=1  Side=Left
  "N " : PMIOPort  Port=2  Side=Left
  wires:
  Ron4/1 -> Breaker3/1
  connections:
  Universal Bridge2/RConn2 -- Parallel RLC Branch/RConn1
  Universal Bridge2/RConn1 -- Parallel RLC Branch/LConn1
  Breaker3/RConn1 -- Universal Bridge2/LConn1
  Universal Bridge2/LConn2 -- "N "/RConn1
  AC/RConn1 -- Breaker3/LConn1

== system Symmetry/Load/Loads/Capacitive_Loads_RST/Capacitive_Load_S/Capacitive_Load_S_1 ==
  Breaker5 : powerlib/Elements/Breaker  InitialState=0  SwitchingTimes="[ 1/60  5/60 ]"  External=on  BreakerResistance=0.01  SnubberResistance=1e7  SnubberCapacitance=inf  Measurements=None  MoreParameters=off  NoBreakLoop=off
  Parallel RLC Branch : powerlib/Elements/Parallel RLC Branch  LConnTagsString=a  RConnTagsString=__new0  BranchType=RC  Resistance=Capacitive_Load_S_RC(1,1)  Inductance=1e-3  SetiL0=off  InitialCurrent=0  Capacitance=Capacitive_Load_S_RC(2,1)  Setx0=off  InitialVoltage=0  Measurements=None
  Ron3 : simulink/Sources/Repeating Sequence Stair  OutValues=Capacitive_Load_S_Switching_Sequence(:,1)  tsamp=Capacitive_Load_S_Switching_Speed(1)  OutMin=[]  OutMax=[]  OutDataTypeStr=float('double')  OutputDataTypeScalingMode=Specify via dialog  OutDataType=float('double')  ConRadixGroup=Best Precision: Vector-wise  OutScaling=2^-12
  Universal Bridge : powerlib/Power Electronics/Universal Bridge  Arms=2  SnubberResistance=1e5  SnubberCapacitance=inf  Device=Diodes  Ron=1e-3  Lon=0  ForwardVoltages="[  0  0  ]"  ForwardVoltage=0.8  GTOparameters=[ 10e-6 , 20e-6 ]  IGBTparameters=[ 1e-6 , 2e-6 ]  Measurements=None  Measurements_2=None  converterType=Rectifier
  AC : PMIOPort  Port=1  Side=Right
  N : PMIOPort  Port=2  Side=Right
  wires:
  Ron3/1 -> Breaker5/1
  connections:
  Universal Bridge/RConn2 -- Parallel RLC Branch/RConn1
  AC/RConn1 -- Breaker5/LConn1
  Universal Bridge/RConn1 -- Parallel RLC Branch/LConn1
  Breaker5/RConn1 -- Universal Bridge/LConn1
  Universal Bridge/LConn2 -- N/RConn1

== system Symmetry/Load/Loads/Capacitive_Loads_RST/Capacitive_Load_S/Capacitive_Load_S_2 ==
  Breaker2 : powerlib/Elements/Breaker  InitialState=0  SwitchingTimes="[ 1/60  5/60 ]"  External=on  BreakerResistance=0.01  SnubberResistance=1e7  SnubberCapacitance=inf  Measurements=None  MoreParameters=off  NoBreakLoop=off
  Parallel RLC Branch : powerlib/Elements/Parallel RLC Branch  LConnTagsString=a  RConnTagsString=__new0  BranchType=RC  Resistance=Capacitive_Load_S_RC(1,2)  Inductance=1e-3  SetiL0=off  InitialCurrent=0  Capacitance=Capacitive_Load_S_RC(2,2)  Setx0=off  InitialVoltage=0  Measurements=None
  Ron1 : simulink/Sources/Repeating Sequence Stair  OutValues=Capacitive_Load_S_Switching_Sequence(:,2)  tsamp=Capacitive_Load_S_Switching_Speed(2)  OutMin=[]  OutMax=[]  OutDataTypeStr=float('double')  OutputDataTypeScalingMode=Specify via dialog  OutDataType=float('double')  ConRadixGroup=Best Precision: Vector-wise  OutScaling=2^-12
  Universal Bridge1 : powerlib/Power Electronics/Universal Bridge  Arms=2  SnubberResistance=1e5  SnubberCapacitance=inf  Device=Diodes  Ron=1e-3  Lon=0  ForwardVoltages="[  0  0  ]"  ForwardVoltage=0.8  GTOparameters=[ 10e-6 , 20e-6 ]  IGBTparameters=[ 1e-6 , 2e-6 ]  Measurements=None  Measurements_2=None  converterType=Rectifier
  AC : PMIOPort  Port=1  Side=Left
  N : PMIOPort  Port=2  Side=Left
  wires:
  Ron1/1 -> Breaker2/1
  connections:
  AC/RConn1 -- Breaker2/LConn1
  Parallel RLC Branch/LConn1 -- Universal Bridge1/RConn1
  Breaker2/RConn1 -- Universal Bridge1/LConn1
  Universal Bridge1/LConn2 -- N/RConn1
  Universal Bridge1/RConn2 -- Parallel RLC Branch/RConn1

== system Symmetry/Load/Loads/Capacitive_Loads_RST/Capacitive_Load_S/Capacitive_Load_S_3 ==
  Breaker3 : powerlib/Elements/Breaker  InitialState=0  SwitchingTimes="[ 1/60  5/60 ]"  External=on  BreakerResistance=0.01  SnubberResistance=1e7  SnubberCapacitance=inf  Measurements=None  MoreParameters=off  NoBreakLoop=off
  Parallel RLC Branch : powerlib/Elements/Parallel RLC Branch  LConnTagsString=a  RConnTagsString=__new0  BranchType=RC  Resistance=Capacitive_Load_S_RC(1,3)  Inductance=1e-3  SetiL0=off  InitialCurrent=0  Capacitance=Capacitive_Load_S_RC(2,3)  Setx0=off  InitialVoltage=0  Measurements=None
  Ron4 : simulink/Sources/Repeating Sequence Stair  OutValues=Capacitive_Load_S_Switching_Sequence(:,3)  tsamp=Capacitive_Load_S_Switching_Speed(3)  OutMin=[]  OutMax=[]  OutDataTypeStr=float('double')  OutputDataTypeScalingMode=Specify via dialog  OutDataType=float('double')  ConRadixGroup=Best Precision: Vector-wise  OutScaling=2^-12
  Universal Bridge2 : powerlib/Power Electronics/Universal Bridge  Arms=2  SnubberResistance=1e5  SnubberCapacitance=inf  Device=Diodes  Ron=1e-3  Lon=0  ForwardVoltages="[  0  0  ]"  ForwardVoltage=0.8  GTOparameters=[ 10e-6 , 20e-6 ]  IGBTparameters=[ 1e-6 , 2e-6 ]  Measurements=None  Measurements_2=None  converterType=Rectifier
  AC : PMIOPort  Port=1  Side=Left
  "N " : PMIOPort  Port=2  Side=Left
  wires:
  Ron4/1 -> Breaker3/1
  connections:
  AC/RConn1 -- Breaker3/LConn1
  Universal Bridge2/LConn2 -- "N "/RConn1
  Breaker3/RConn1 -- Universal Bridge2/LConn1
  Universal Bridge2/RConn1 -- Parallel RLC Branch/LConn1
  Universal Bridge2/RConn2 -- Parallel RLC Branch/RConn1

== system Symmetry/Load/Loads/Capacitive_Loads_RST/Capacitive_Load_T/Capacitive_Load_R_1 ==
  Breaker5 : powerlib/Elements/Breaker  InitialState=0  SwitchingTimes="[ 1/60  5/60 ]"  External=on  BreakerResistance=0.01  SnubberResistance=1e7  SnubberCapacitance=inf  Measurements=None  MoreParameters=off  NoBreakLoop=off
  Parallel RLC Branch : powerlib/Elements/Parallel RLC Branch  LConnTagsString=a  RConnTagsString=__new0  BranchType=RC  Resistance=Capacitive_Load_T_RC(1,1)  Inductance=1e-3  SetiL0=off  InitialCurrent=0  Capacitance=Capacitive_Load_T_RC(2,1)  Setx0=off  InitialVoltage=0  Measurements=None
  Ron3 : simulink/Sources/Repeating Sequence Stair  OutValues=Capacitive_Load_T_Switching_Sequence(:,1)  tsamp=Capacitive_Load_T_Switching_Speed(1)  OutMin=[]  OutMax=[]  OutDataTypeStr=float('double')  OutputDataTypeScalingMode=Specify via dialog  OutDataType=float('double')  ConRadixGroup=Best Precision: Vector-wise  OutScaling=2^-12
  Universal Bridge : powerlib/Power Electronics/Universal Bridge  Arms=2  SnubberResistance=1e5  SnubberCapacitance=inf  Device=Diodes  Ron=1e-3  Lon=0  ForwardVoltages="[  0  0  ]"  ForwardVoltage=0.8  GTOparameters=[ 10e-6 , 20e-6 ]  IGBTparameters=[ 1e-6 , 2e-6 ]  Measurements=None  Measurements_2=None  converterType=Rectifier
  AC : PMIOPort  Port=1  Side=Right
  N : PMIOPort  Port=2  Side=Right
  wires:
  Ron3/1 -> Breaker5/1
  connections:
  Universal Bridge/LConn2 -- N/RConn1
  Breaker5/RConn1 -- Universal Bridge/LConn1
  Universal Bridge/RConn1 -- Parallel RLC Branch/LConn1
  AC/RConn1 -- Breaker5/LConn1
  Universal Bridge/RConn2 -- Parallel RLC Branch/RConn1

== system Symmetry/Load/Loads/Capacitive_Loads_RST/Capacitive_Load_T/Capacitive_Load_R_2 ==
  Breaker2 : powerlib/Elements/Breaker  InitialState=0  SwitchingTimes="[ 1/60  5/60 ]"  External=on  BreakerResistance=0.01  SnubberResistance=1e7  SnubberCapacitance=inf  Measurements=None  MoreParameters=off  NoBreakLoop=off
  Parallel RLC Branch : powerlib/Elements/Parallel RLC Branch  LConnTagsString=a  RConnTagsString=__new0  BranchType=RC  Resistance=Capacitive_Load_T_RC(1,2)  Inductance=1e-3  SetiL0=off  InitialCurrent=0  Capacitance=Capacitive_Load_T_RC(2,2)  Setx0=off  InitialVoltage=0  Measurements=None
  Ron1 : simulink/Sources/Repeating Sequence Stair  OutValues=Capacitive_Load_T_Switching_Sequence(:,2)  tsamp=Capacitive_Load_T_Switching_Speed(2)  OutMin=[]  OutMax=[]  OutDataTypeStr=float('double')  OutputDataTypeScalingMode=Specify via dialog  OutDataType=float('double')  ConRadixGroup=Best Precision: Vector-wise  OutScaling=2^-12
  Universal Bridge1 : powerlib/Power Electronics/Universal Bridge  Arms=2  SnubberResistance=1e5  SnubberCapacitance=inf  Device=Diodes  Ron=1e-3  Lon=0  ForwardVoltages="[  0  0  ]"  ForwardVoltage=0.8  GTOparameters=[ 10e-6 , 20e-6 ]  IGBTparameters=[ 1e-6 , 2e-6 ]  Measurements=None  Measurements_2=None  converterType=Rectifier
  AC : PMIOPort  Port=1  Side=Left
  N : PMIOPort  Port=2  Side=Left
  wires:
  Ron1/1 -> Breaker2/1
  connections:
  Universal Bridge1/RConn2 -- Parallel RLC Branch/RConn1
  Universal Bridge1/LConn2 -- N/RConn1
  Breaker2/RConn1 -- Universal Bridge1/LConn1
  Parallel RLC Branch/LConn1 -- Universal Bridge1/RConn1
  AC/RConn1 -- Breaker2/LConn1

== system Symmetry/Load/Loads/Capacitive_Loads_RST/Capacitive_Load_T/Capacitive_Load_R_3 ==
  Breaker3 : powerlib/Elements/Breaker  InitialState=0  SwitchingTimes="[ 1/60  5/60 ]"  External=on  BreakerResistance=0.01  SnubberResistance=1e7  SnubberCapacitance=inf  Measurements=None  MoreParameters=off  NoBreakLoop=off
  Parallel RLC Branch : powerlib/Elements/Parallel RLC Branch  LConnTagsString=a  RConnTagsString=__new0  BranchType=RC  Resistance=Capacitive_Load_T_RC(1,3)  Inductance=1e-3  SetiL0=off  InitialCurrent=0  Capacitance=Capacitive_Load_T_RC(2,3)  Setx0=off  InitialVoltage=0  Measurements=None
  Ron4 : simulink/Sources/Repeating Sequence Stair  OutValues=Capacitive_Load_T_Switching_Sequence(:,3)  tsamp=Capacitive_Load_T_Switching_Speed(3)  OutMin=[]  OutMax=[]  OutDataTypeStr=float('double')  OutputDataTypeScalingMode=Specify via dialog  OutDataType=float('double')  ConRadixGroup=Best Precision: Vector-wise  OutScaling=2^-12
  Universal Bridge2 : powerlib/Power Electronics/Universal Bridge  Arms=2  SnubberResistance=1e5  SnubberCapacitance=inf  Device=Diodes  Ron=1e-3  Lon=0  ForwardVoltages="[  0  0  ]"  ForwardVoltage=0.8  GTOparameters=[ 10e-6 , 20e-6 ]  IGBTparameters=[ 1e-6 , 2e-6 ]  Measurements=None  Measurements_2=None  converterType=Rectifier
  AC : PMIOPort  Port=1  Side=Left
  "N " : PMIOPort  Port=2  Side=Left
  wires:
  Ron4/1 -> Breaker3/1
  connections:
  Universal Bridge2/RConn2 -- Parallel RLC Branch/RConn1
  Universal Bridge2/RConn1 -- Parallel RLC Branch/LConn1
  Breaker3/RConn1 -- Universal Bridge2/LConn1
  Universal Bridge2/LConn2 -- "N "/RConn1
  AC/RConn1 -- Breaker3/LConn1
